simulink model "PassengerCar"  (R2019b)
settings: Solver=ode1  StartTime=0  StopTime=25  FixedStep=1.0000000000000000e-003  RelTol=1e-3
InitFcn:
  | sampleTime = str2double(get_param(bdroot, 'FixedStep'));
undefined symbols (not defined in the file or in its folder): AccPedalPos, BrakePedalPos, BrakeSwitch, DiscIntNeverNeededParam, DYNA4, EngSpd, IgnitionSwitch, InitialGear, InitialSpeed, IntendedEngTrq, LeftIndicator, MainBrakePress, MaxGear, MDL, MinGear, RefAcc, RefLane, RefLatPos, RefPath, RefPathCurv, RefSpd, RefSpdPreview, RefSpdRetrospect, RightIndicator, SteeringWheelAng, SteeringWheelTrq, UserDefinedRefValue, vm_const
libraries: UtilitiesLibrary x31, simulink x18, WheelSystemModules x13, LongitudinalControllerModules x13, LateralControllerModules x7, AnimationBusselectorModules x5, EnvironmentModules x5, BasicEngineControlModules x5, MiscellaneousControlModules x5, Animation3Modules x4, AuxiliariesModules x4, TireModules x4
(part 30 of 39)

== system PassengerCar/Vehicle/Drivetrain/DrivetrainPhysics/DrivetrainPhysicsInputs/InputFromWheelSystem ==
  fromWheelSystem : Inport
  TDBusSelector : BusSelector  OutputSignals=FrontLeft.Wheel.RotSpd[rad/s],FrontRight.Wheel.RotSpd[rad/s],RearLeft.Wheel.RotSpd[rad/s],RearRight.Wheel.RotSpd[rad/s],Rear2Left.Wheel.RotSpd[rad/s],Rear2Right.Wheel.RotSpd[rad/s],Rear3Left.Wheel.RotSpd[rad/s],Rear3Right.Wheel.RotSpd[rad/s]
  __TDD__WheelSystem.RotSpdFL[rad/s] : Demux  Outputs=[1]
  __TDD__WheelSystem.RotSpdFR[rad/s] : Demux  Outputs=[1]
  __TDD__WheelSystem.RotSpdR2L[rad/s] : Demux  Outputs=[1]
  __TDD__WheelSystem.RotSpdR2R[rad/s] : Demux  Outputs=[1]
  __TDD__WheelSystem.RotSpdR3L[rad/s] : Demux  Outputs=[1]
  __TDD__WheelSystem.RotSpdR3R[rad/s] : Demux  Outputs=[1]
  __TDD__WheelSystem.RotSpdRL[rad/s] : Demux  Outputs=[1]
  __TDD__WheelSystem.RotSpdRR[rad/s] : Demux  Outputs=[1]
  __TDO__WheelSystem : BusCreator  Inputs=8
  WheelSystem___UNIQUE_1 : Outport  Description=|  PortDimensions=[8]  VectorParamsAs1DForOutWhenUnconnected=off
      | <name>FrontLeft.Wheel.RotSpd[rad/s]</name>
      | <comment></comment>
  wires:
  fromWheelSystem/1 -> TDBusSelector/1
  TDBusSelector/1 -> __TDD__WheelSystem.RotSpdFL[rad/s]/1  "<RotSpd[rad/s]>"
  __TDD__WheelSystem.RotSpdFL[rad/s]/1 -> __TDO__WheelSystem/1  "RotSpdFL[rad/s]"
  TDBusSelector/2 -> __TDD__WheelSystem.RotSpdFR[rad/s]/1  "<RotSpd[rad/s]>"
  __TDD__WheelSystem.RotSpdFR[rad/s]/1 -> __TDO__WheelSystem/2  "RotSpdFR[rad/s]"
  TDBusSelector/3 -> __TDD__WheelSystem.RotSpdRL[rad/s]/1  "<RotSpd[rad/s]>"
  __TDD__WheelSystem.RotSpdRL[rad/s]/1 -> __TDO__WheelSystem/3  "RotSpdRL[rad/s]"
  TDBusSelector/4 -> __TDD__WheelSystem.RotSpdRR[rad/s]/1  "<RotSpd[rad/s]>"
  __TDD__WheelSystem.RotSpdRR[rad/s]/1 -> __TDO__WheelSystem/4  "RotSpdRR[rad/s]"
  TDBusSelector/5 -> __TDD__WheelSystem.RotSpdR2L[rad/s]/1  "<RotSpd[rad/s]>"
  __TDD__WheelSystem.RotSpdR2L[rad/s]/1 -> __TDO__WheelSystem/5  "RotSpdR2L[rad/s]"
  TDBusSelector/6 -> __TDD__WheelSystem.RotSpdR2R[rad/s]/1  "<RotSpd[rad/s]>"
  __TDD__WheelSystem.RotSpdR2R[rad/s]/1 -> __TDO__WheelSystem/6  "RotSpdR2R[rad/s]"
  TDBusSelector/7 -> __TDD__WheelSystem.RotSpdR3L[rad/s]/1  "<RotSpd[rad/s]>"
  __TDD__WheelSystem.RotSpdR3L[rad/s]/1 -> __TDO__WheelSystem/7  "RotSpdR3L[rad/s]"
  TDBusSelector/8 -> __TDD__WheelSystem.RotSpdR3R[rad/s]/1  "<RotSpd[rad/s]>"
  __TDD__WheelSystem.RotSpdR3R[rad/s]/1 -> __TDO__WheelSystem/8  "RotSpdR3R[rad/s]"
  __TDO__WheelSystem/1 -> WheelSystem___UNIQUE_1/1  "WheelSystem"

== system PassengerCar/Vehicle/Drivetrain/DrivetrainPhysics/DrivetrainPhysicsOutputs/ClutchOutput ==
  note: negative clutch torque accelerates driven plate
  ClutchStates : Inport
  ClutchOutput : Subsystem  Tag=TESIS DYNAware Interface Block  mask{NeedsUpdate=off, SignalInfo=|}
      mask SignalInfo=|
      | {
      |   "Version": "4.6",
      |   "MuxedOutputBusName": "Clutch",
      |   "MuxedInputBusName": "input",
      |   "MuxedInputSelected": false,
      |   "MuxedOutputSelected": true,
      |   "SignalData": [
      |     {
      |       "initialValue": "0.0",
      |       "name": "Trq[Nm]",
      |       "comment": "",
      |       "minString": "",
      |       "maxString": "",
      |       "width": 1,
      |       "dataType": 0,
      |       "signalType": 0,
      |       "createSignal": false,
      |       "outputName": "Trq[Nm]",
      |       "generateSignalAccessBlock": false,
      |       "accessId": "$(parentId).$(blockName).$(outputName)"
      |     },
      |     {
      |       "initialValue": "0.0",
      |       "name": "Pos[0_1]",
      |       "comment": "",
      |       "minString": "",
      |       "maxString": "",
      |       "width": 1,
      |       "dataType": 0,
      |       "signalType": 0,
      |       "createSignal": false,
      |       "outputName": "Pos[0_1]",
      |       "generateSignalAccessBlock": false,
      |       "accessId": "$(parentId).$(blockName).$(outputName)"
      |     }
      |   ]
      | }
      mask prompts: NeedsUpdate "Specify, if subsystem content needs to be updated"; SignalInfo "Signal Info (json)"
      mask help: DYNA4 Interface Block Version 4.6
      mask init:
      | blockName = get_param(gcbh, 'Name');
      | parentId = DYNA4.ModelHandling.AccessID.getFromHierarchy(gcbh);
      | TD.InterfaceBlock.ModelCallbacks.GenerateContent(gcb);
      settings: DeleteFcn=TD.InterfaceBlock.ModelCallbacks.CloseGUI( gcbh );  NameChangeFcn=TD.InterfaceBlock.ModelCallbacks.BlockRenamedHandler(gcbh);  OpenFcn=TD.InterfaceBlock.ModelCallbacks.OpenGUI( gcbh );  CloseFcn=TD.InterfaceBlock.ModelCallbacks.CloseGUI( gcbh );
      mask Display:
      | image('InterfaceBlock.png','center');
      | port_label('input',1, 'Trq[Nm]');
      | port_label('input',2, 'Pos[0_1]');
      | port_label('output',1, 'Clutch');
  Demux2 : Demux  Outputs=[1 1]
  Clutch : Outport  VectorParamsAs1DForOutWhenUnconnected=off
  wires:
  Demux2/2 -> ClutchOutput/2(Pos[0_1]___UNIQUE_1)
  ClutchStates/1 -> Demux2/1
  ClutchOutput/1(Clutch___UNIQUE_1) -> Clutch/1
  Demux2/1 -> ClutchOutput/1(Trq[Nm]___UNIQUE_1)

== system PassengerCar/Vehicle/Drivetrain/DrivetrainPhysics/DrivetrainPhysicsOutputs/DrivetrainPhysicsOutput ==
  EngSpd[rad/s]___UNIQUE_1 : Inport  Description=|  PortDimensions=[1]
      | <name>EngSpd[rad/s]</name>
      | <comment></comment>
  EngAcc[rad/s**2]___UNIQUE_1 : Inport  Description=|  Port=2  PortDimensions=[1]
      | <name>EngAcc[rad/s**2]</name>
      | <comment></comment>
  Clutch___UNIQUE_1 : Inport  Description=|  Port=3
      | <name>Clutch</name>
      | <comment></comment>
  Transmission___UNIQUE_1 : Inport  Description=|  Port=4
      | <name>Transmission</name>
      | <comment></comment>
  TransferCase___UNIQUE_1 : Inport  Description=|  Port=5
      | <name>TransferCase</name>
      | <comment></comment>
  FrontDifferential___UNIQUE_1 : Inport  Description=|  Port=6
      | <name>FrontDifferential</name>
      | <comment></comment>
  FrontLeftShaft___UNIQUE_1 : Inport  Description=|  Port=7
      | <name>FrontLeftShaft</name>
      | <comment></comment>
  FrontRightShaft___UNIQUE_1 : Inport  Description=|  Port=8
      | <name>FrontRightShaft</name>
      | <comment></comment>
  RearDifferential___UNIQUE_1 : Inport  Description=|  Port=9
      | <name>RearDifferential</name>
      | <comment></comment>
  RearLeftShaft___UNIQUE_1 : Inport  Description=|  Port=10
      | <name>RearLeftShaft</name>
      | <comment></comment>
  RearRightShaft___UNIQUE_1 : Inport  Description=|  Port=11
      | <name>RearRightShaft</name>
      | <comment></comment>
  Rear2Differential___UNIQUE_1 : Inport  Description=|  Port=12
      | <name>Rear2Differential</name>
      | <comment></comment>
  Rear2LeftShaft___UNIQUE_1 : Inport  Description=|  Port=13
      | <name>Rear2LeftShaft</name>
      | <comment></comment>
  Rear2RightShaft___UNIQUE_1 : Inport  Description=|  Port=14
      | <name>Rear2RightShaft</name>
      | <comment></comment>
  Rear3Differential___UNIQUE_1 : Inport  Description=|  Port=15
      | <name>Rear3Differential</name>
      | <comment></comment>
  Rear3LeftShaft___UNIQUE_1 : Inport  Description=|  Port=16
      | <name>Rear3LeftShaft</name>
      | <comment></comment>
  Rear3RightShaft___UNIQUE_1 : Inport  Description=|  Port=17
      | <name>Rear3RightShaft</name>
      | <comment></comment>
  TotalRatio[-]___UNIQUE_1 : Inport  Description=|  Port=18  PortDimensions=[1]
      | <name>TotalRatio[-]</name>
      | <comment></comment>
  __TDD__DrivetrainPhysics.EngAcc[rad/s**2] : Demux  Outputs=[1]
  __TDD__DrivetrainPhysics.EngSpd[rad/s] : Demux  Outputs=[1]
  __TDD__DrivetrainPhysics.TotalRatio[-] : Demux  Outputs=[1]
  __TDO__DrivetrainPhysics : BusCreator  Inputs=18
  DrivetrainPhysics___UNIQUE_1 : Outport  Description=|  VectorParamsAs1DForOutWhenUnconnected=off
      | <name>EngSpd[rad/s]</name>
      | <comment></comment>
  wires:
  EngSpd[rad/s]___UNIQUE_1/1 -> __TDD__DrivetrainPhysics.EngSpd[rad/s]/1
  __TDD__DrivetrainPhysics.EngSpd[rad/s]/1 -> __TDO__DrivetrainPhysics/1  "EngSpd[rad/s]"
  EngAcc[rad/s**2]___UNIQUE_1/1 -> __TDD__DrivetrainPhysics.EngAcc[rad/s**2]/1
  __TDD__DrivetrainPhysics.EngAcc[rad/s**2]/1 -> __TDO__DrivetrainPhysics/2  "EngAcc[rad/s**2]"
  Clutch___UNIQUE_1/1 -> __TDO__DrivetrainPhysics/3  "Clutch"
  Transmission___UNIQUE_1/1 -> __TDO__DrivetrainPhysics/4  "Transmission"
  TransferCase___UNIQUE_1/1 -> __TDO__DrivetrainPhysics/5  "TransferCase"
  FrontDifferential___UNIQUE_1/1 -> __TDO__DrivetrainPhysics/6  "FrontDifferential"
  FrontLeftShaft___UNIQUE_1/1 -> __TDO__DrivetrainPhysics/7  "FrontLeftShaft"
  FrontRightShaft___UNIQUE_1/1 -> __TDO__DrivetrainPhysics/8  "FrontRightShaft"
  RearDifferential___UNIQUE_1/1 -> __TDO__DrivetrainPhysics/9  "RearDifferential"
  RearLeftShaft___UNIQUE_1/1 -> __TDO__DrivetrainPhysics/10  "RearLeftShaft"
  RearRightShaft___UNIQUE_1/1 -> __TDO__DrivetrainPhysics/11  "RearRightShaft"
  Rear2Differential___UNIQUE_1/1 -> __TDO__DrivetrainPhysics/12  "Rear2Differential"
  Rear2LeftShaft___UNIQUE_1/1 -> __TDO__DrivetrainPhysics/13  "Rear2LeftShaft"
  Rear2RightShaft___UNIQUE_1/1 -> __TDO__DrivetrainPhysics/14  "Rear2RightShaft"
  Rear3Differential___UNIQUE_1/1 -> __TDO__DrivetrainPhysics/15  "Rear3Differential"
  Rear3LeftShaft___UNIQUE_1/1 -> __TDO__DrivetrainPhysics/16  "Rear3LeftShaft"
  Rear3RightShaft___UNIQUE_1/1 -> __TDO__DrivetrainPhysics/17  "Rear3RightShaft"
  TotalRatio[-]___UNIQUE_1/1 -> __TDD__DrivetrainPhysics.TotalRatio[-]/1
  __TDD__DrivetrainPhysics.TotalRatio[-]/1 -> __TDO__DrivetrainPhysics/18  "TotalRatio[-]"
  __TDO__DrivetrainPhysics/1 -> DrivetrainPhysics___UNIQUE_1/1  "DrivetrainPhysics"

== system PassengerCar/Vehicle/Drivetrain/DrivetrainPhysics/DrivetrainPhysicsOutputs/FrontDifferentialOutput ==
  In2 : Inport
  FrontDifferentialOutput : Subsystem  Tag=TESIS DYNAware Interface Block  mask{NeedsUpdate=off, SignalInfo=|}
      mask SignalInfo=|
      | {
      |   "Version": "4.6",
      |   "MuxedOutputBusName": "FrontDifferential",
      |   "MuxedInputBusName": "",
      |   "MuxedInputSelected": false,
      |   "MuxedOutputSelected": true,
      |   "SignalData": [
      |     {
      |       "initialValue": "0.0",
      |       "name": "InSpd[rad/s]",
      |       "comment": "",
      |       "minString": "",
      |       "maxString": "",
      |       "width": 1,
      |       "dataType": 0,
      |       "signalType": 0,
      |       "createSignal": false,
      |       "outputName": "InSpd[rad/s]",
      |       "generateSignalAccessBlock": false,
      |       "accessId": "$(parentId).$(blockName).$(outputName)"
      |     },
      |     {
      |       "initialValue": "0.0",
      |       "name": "LeftOutCutTrq[Nm]",
      |       "comment": "",
      |       "minString": "",
      |       "maxString": "",
      |       "width": 1,
      |       "dataType": 0,
      |       "signalType": 0,
      |       "createSignal": false,
      |       "outputName": "LeftOutCutTrq[Nm]",
      |       "generateSignalAccessBlock": false,
      |       "accessId": "$(parentId).$(blockName).$(outputName)"
      |     },
      |     {
      |       "initialValue": "0.0",
      |       "name": "RightOutCutTrq[Nm]",
      |       "comment": "",
      |       "minString": "",
      |       "maxString": "",
      |       "width": 1,
      |       "dataType": 0,
      |       "signalType": 0,
      |       "createSignal": false,
      |       "outputName": "RightOutCutTrq[Nm]",
      |       "generateSignalAccessBlock": false,
      |       "accessId": "$(parentId).$(blockName).$(outputName)"
      |     },
      |     {
      |       "initialValue": "0.0",
      |       "name": "LossPower[W]",
      |       "comment": "",
      |       "minString": "",
      |       "maxString": "",
      |       "width": 1,
      |       "dataType": 0,
      |       "signalType": 0,
      |       "createSignal": false,
      |       "outputName": "LossPower[W]",
      |       "generateSignalAccessBlock": false,
      |       "accessId": "$(parentId).$(blockName).$(outputName)"
      |     }
      |   ]
      | }
      mask prompts: NeedsUpdate "Specify, if subsystem content needs to be updated"; SignalInfo "Signal Info (json)"
      mask help: DYNA4 Interface Block Version 4.6
      mask init:
      | blockName = get_param(gcbh, 'Name');
      | parentId = DYNA4.ModelHandling.AccessID.getFromHierarchy(gcbh);
      | TD.InterfaceBlock.ModelCallbacks.GenerateContent(gcb);
      settings: DeleteFcn=TD.InterfaceBlock.ModelCallbacks.CloseGUI( gcbh );  NameChangeFcn=TD.InterfaceBlock.ModelCallbacks.BlockRenamedHandler(gcbh);  OpenFcn=TD.InterfaceBlock.ModelCallbacks.OpenGUI( gcbh );  CloseFcn=TD.InterfaceBlock.ModelCallbacks.CloseGUI( gcbh );
      mask Display:
      | image('InterfaceBlock.png','center');
      | port_label('input',1, 'InSpd[rad/s]');
      | port_label('input',2, 'LeftOutCutTrq[Nm]');
      | port_label('input',3, 'RightOutCutTrq[Nm]');
      | port_label('input',4, 'LossPower[W]');
      | port_label('output',1, 'FrontDifferential');
  zero : Constant  Value=0
  zero1 : Constant  Value=0
  zero2 : Constant  Value=0
  FrontDifferential : Outport  VectorParamsAs1DForOutWhenUnconnected=off
  wires:
  In2/1 -> FrontDifferentialOutput/1(InSpd[rad/s]___UNIQUE_1)
  FrontDifferentialOutput/1(FrontDifferential___UNIQUE_1) -> FrontDifferential/1
  zero/1 -> FrontDifferentialOutput/2(LeftOutCutTrq[Nm]___UNIQUE_1)
  zero2/1 -> FrontDifferentialOutput/4(LossPower[W]___UNIQUE_1)
  zero1/1 -> FrontDifferentialOutput/3(RightOutCutTrq[Nm]___UNIQUE_1)

== system PassengerCar/Vehicle/Drivetrain/DrivetrainPhysics/DrivetrainPhysicsOutputs/FrontLeftShaftOutput ==
  In1 : Inport
  Demux : Demux  Outputs=[1 1 1 1 1]
  FrontLeftShaftOutput : Subsystem  Tag=TESIS DYNAware Interface Block  mask{NeedsUpdate=off, SignalInfo=|}
      mask SignalInfo=|
      | {
      |   "Version": "4.6",
      |   "MuxedOutputBusName": "FrontLeftShaft",
      |   "MuxedInputBusName": "input",
      |   "MuxedInputSelected": false,
      |   "MuxedOutputSelected": true,
      |   "SignalData": [
      |     {
      |       "initialValue": "0.0",
      |       "name": "Trq[Nm]",
      |       "comment": "",
      |       "minString": "",
      |       "maxString": "",
      |       "width": 1,
      |       "dataType": 0,
      |       "signalType": 0,
      |       "createSignal": false,
      |       "outputName": "Trq[Nm]",
      |       "generateSignalAccessBlock": false,
      |       "accessId": "$(parentId).$(blockName).$(outputName)"
      |     },
      |     {
      |       "initialValue": "0.0",
      |       "name": "RotSpdDifferentialOut[rad/s]",
      |       "comment": "",
      |       "minString": "",
      |       "maxString": "",
      |       "width": 1,
      |       "dataType": 0,
      |       "signalType": 0,
      |       "createSignal": false,
      |       "outputName": "RotSpdDifferentialOut[rad/s]",
      |       "generateSignalAccessBlock": false,
      |       "accessId": "$(parentId).$(blockName).$(outputName)"
      |     },
      |     {
      |       "initialValue": "0.0",
      |       "name": "RotAcc[rad/s**2]",
      |       "comment": "",
      |       "minString": "",
      |       "maxString": "",
      |       "width": 1,
      |       "dataType": 0,
      |       "signalType": 0,
      |       "createSignal": false,
      |       "outputName": "RotAcc[rad/s**2]",
      |       "generateSignalAccessBlock": false,
      |       "accessId": "$(parentId).$(blockName).$(outputName)"
      |     },
      |     {
      |       "initialValue": "0.0",
      |       "name": "DerivativeOfTrq_wrt_RotAng[Nm/rad]",
      |       "comment": "",
      |       "minString": "",
      |       "maxString": "",
      |       "width": 1,
      |       "dataType": 0,
      |       "signalType": 0,
      |       "createSignal": false,
      |       "outputName": "DerivativeOfTrq_wrt_RotAng[Nm/rad]",
      |       "generateSignalAccessBlock": false,
      |       "accessId": "$(parentId).$(blockName).$(outputName)"
      |     },
      |     {
      |       "initialValue": "0.0",
      |       "name": "DerivativeOfTrq_wrt_WheelSpd[Nm/(rad/s)]",
      |       "comment": "",
      |       "minString": "",
      |       "maxString": "",
      |       "width": 1,
      |       "dataType": 0,
      |       "signalType": 0,
      |       "createSignal": false,
      |       "outputName": "DerivativeOfTrq_wrt_WheelSpd[Nm/(rad/s)]",
      |       "generateSignalAccessBlock": false,
      |       "accessId": "$(parentId).$(blockName).$(outputName)"
      |     },
      |     {
      |       "initialValue": "0.0",
      |       "name": "AddInrt[kg*m**2]",
      |       "comment": "",
      |       "minString": "",
      |       "maxString": "",
      |       "width": 1,
      |       "dataType": 0,
      |       "signalType": 0,
      |       "createSignal": false,
      |       "outputName": "AddInrt[kg*m**2]",
      |       "generateSignalAccessBlock": false,
      |       "accessId": "$(parentId).$(blockName).$(outputName)"
      |     },
      |     {
      |       "initialValue": "0.0",
      |       "name": "FrictionTrq[Nm]",
      |       "comment": "",
      |       "minString": "",
      |       "maxString": "",
      |       "width": 1,
      |       "dataType": 0,
      |       "signalType": 0,
      |       "createSignal": false,
      |       "outputName": "FrictionTrq[Nm]",
      |       "generateSignalAccessBlock": false,
      |       "accessId": "$(parentId).$(blockName).$(outputName)"
      |     }
      |   ]
      | }
      mask prompts: NeedsUpdate "Specify, if subsystem content needs to be updated"; SignalInfo "Signal Info (json)"
      mask help: DYNA4 Interface Block Version 4.6
      mask init:
      | blockName = get_param(gcbh, 'Name');
      | parentId = DYNA4.ModelHandling.AccessID.getFromHierarchy(gcbh);
      | TD.InterfaceBlock.ModelCallbacks.GenerateContent(gcb);
      settings: DeleteFcn=TD.InterfaceBlock.ModelCallbacks.CloseGUI( gcbh );  NameChangeFcn=TD.InterfaceBlock.ModelCallbacks.BlockRenamedHandler(gcbh);  OpenFcn=TD.InterfaceBlock.ModelCallbacks.OpenGUI( gcbh );  CloseFcn=TD.InterfaceBlock.ModelCallbacks.CloseGUI( gcbh );
      mask Display:
      | image('InterfaceBlock.png','center');
      | port_label('input',1, 'Trq[Nm]');
      | port_label('input',2, 'RotSpdDifferentialOut[rad/s]');
      | port_label('input',3, 'RotAcc[rad/s**2]');
      | port_label('input',4, 'DerivativeOfTrq_wrt_RotAng[Nm/rad]');
      | port_label('input',5, 'DerivativeOfTrq_wrt_WheelSpd[Nm/(rad/s)]');
      | port_label('input',6, 'AddInrt[kg*m**2]');
      | port_label('input',7, 'FrictionTrq[Nm]');
      | port_label('output',1, 'FrontLeftShaft');
  zero : Constant  Value=0
  zero1 : Constant  Value=0
  FrontLeftShaft : Outport  VectorParamsAs1DForOutWhenUnconnected=off
  wires:
  In1/1 -> Demux/1
  FrontLeftShaftOutput/1(FrontLeftShaft___UNIQUE_1) -> FrontLeftShaft/1
  Demux/3 -> FrontLeftShaftOutput/3(RotAcc[rad/s**2]___UNIQUE_1)
  zero1/1 -> FrontLeftShaftOutput/7(FrictionTrq[Nm]___UNIQUE_1)
  zero/1 -> FrontLeftShaftOutput/6(AddInrt[kg*m**2]___UNIQUE_1)
  Demux/5 -> FrontLeftShaftOutput/5(DerivativeOfTrq_wrt_WheelSpd[Nm/(rad/s)]___UNIQUE_1)
  Demux/4 -> FrontLeftShaftOutput/4(DerivativeOfTrq_wrt_RotAng[Nm/rad]___UNIQUE_1)
  Demux/2 -> FrontLeftShaftOutput/2(RotSpdDifferentialOut[rad/s]___UNIQUE_1)
  Demux/1 -> FrontLeftShaftOutput/1(Trq[Nm]___UNIQUE_1)

== system PassengerCar/Vehicle/Drivetrain/DrivetrainPhysics/DrivetrainPhysicsOutputs/FrontRightShaftOutput ==
  In1 : Inport
  Demux : Demux  Outputs=[1 1 1 1 1]
  FrontRightShaftOutput : Subsystem  Tag=TESIS DYNAware Interface Block  mask{NeedsUpdate=off, SignalInfo=|}
      mask SignalInfo=|
      | {
      |   "Version": "4.6",
      |   "MuxedOutputBusName": "FrontRightShaft",
      |   "MuxedInputBusName": "input",
      |   "MuxedInputSelected": false,
      |   "MuxedOutputSelected": true,
      |   "SignalData": [
      |     {
      |       "initialValue": "0.0",
      |       "name": "Trq[Nm]",
      |       "comment": "",
      |       "minString": "",
      |       "maxString": "",
      |       "width": 1,
      |       "dataType": 0,
      |       "signalType": 0,
      |       "createSignal": false,
      |       "outputName": "Trq[Nm]",
      |       "generateSignalAccessBlock": false,
      |       "accessId": "$(parentId).$(blockName).$(outputName)"
      |     },
      |     {
      |       "initialValue": "0.0",
      |       "name": "RotSpdDifferentialOut[rad/s]",
      |       "comment": "",
      |       "minString": "",
      |       "maxString": "",
      |       "width": 1,
      |       "dataType": 0,
      |       "signalType": 0,
      |       "createSignal": false,
      |       "outputName": "RotSpdDifferentialOut[rad/s]",
      |       "generateSignalAccessBlock": false,
      |       "accessId": "$(parentId).$(blockName).$(outputName)"
      |     },
      |     {
      |       "initialValue": "0.0",
      |       "name": "RotAcc[rad/s**2]",
      |       "comment": "",
      |       "minString": "",
      |       "maxString": "",
      |       "width": 1,
      |       "dataType": 0,
      |       "signalType": 0,
      |       "createSignal": false,
      |       "outputName": "RotAcc[rad/s**2]",
      |       "generateSignalAccessBlock": false,
      |       "accessId": "$(parentId).$(blockName).$(outputName)"
      |     },
      |     {
      |       "initialValue": "0.0",
      |       "name": "DerivativeOfTrq_wrt_RotAng[Nm/rad]",
      |       "comment": "",
      |       "minString": "",
      |       "maxString": "",
      |       "width": 1,
      |       "dataType": 0,
      |       "signalType": 0,
      |       "createSignal": false,
      |       "outputName": "DerivativeOfTrq_wrt_RotAng[Nm/rad]",
      |       "generateSignalAccessBlock": false,
      |       "accessId": "$(parentId).$(blockName).$(outputName)"
      |     },
      |     {
      |       "initialValue": "0.0",
      |       "name": "DerivativeOfTrq_wrt_WheelSpd[Nm/(rad/s)]",
      |       "comment": "",
      |       "minString": "",
      |       "maxString": "",
      |       "width": 1,
      |       "dataType": 0,
      |       "signalType": 0,
      |       "createSignal": false,
      |       "outputName": "DerivativeOfTrq_wrt_WheelSpd[Nm/(rad/s)]",
      |       "generateSignalAccessBlock": false,
      |       "accessId": "$(parentId).$(blockName).$(outputName)"
      |     },
      |     {
      |       "initialValue": "0.0",
      |       "name": "AddInrt[kg*m**2]",
      |       "comment": "",
      |       "minString": "",
      |       "maxString": "",
      |       "width": 1,
      |       "dataType": 0,
      |       "signalType": 0,
      |       "createSignal": false,
      |       "outputName": "AddInrt[kg*m**2]",
      |       "generateSignalAccessBlock": false,
      |       "accessId": "$(parentId).$(blockName).$(outputName)"
      |     },
      |     {
      |       "initialValue": "0.0",
      |       "name": "FrictionTrq[Nm]",
      |       "comment": "",
      |       "minString": "",
      |       "maxString": "",
      |       "width": 1,
      |       "dataType": 0,
      |       "signalType": 0,
      |       "createSignal": false,
      |       "outputName": "FrictionTrq[Nm]",
      |       "generateSignalAccessBlock": false,
      |       "accessId": "$(parentId).$(blockName).$(outputName)"
      |     }
      |   ]
      | }
      mask prompts: NeedsUpdate "Specify, if subsystem content needs to be updated"; SignalInfo "Signal Info (json)"
      mask help: DYNA4 Interface Block Version 4.6
      mask init:
      | blockName = get_param(gcbh, 'Name');
      | parentId = DYNA4.ModelHandling.AccessID.getFromHierarchy(gcbh);
      | TD.InterfaceBlock.ModelCallbacks.GenerateContent(gcb);
      settings: DeleteFcn=TD.InterfaceBlock.ModelCallbacks.CloseGUI( gcbh );  NameChangeFcn=TD.InterfaceBlock.ModelCallbacks.BlockRenamedHandler(gcbh);  OpenFcn=TD.InterfaceBlock.ModelCallbacks.OpenGUI( gcbh );  CloseFcn=TD.InterfaceBlock.ModelCallbacks.CloseGUI( gcbh );
      mask Display:
      | image('InterfaceBlock.png','center');
      | port_label('input',1, 'Trq[Nm]');
      | port_label('input',2, 'RotSpdDifferentialOut[rad/s]');
      | port_label('input',3, 'RotAcc[rad/s**2]');
      | port_label('input',4, 'DerivativeOfTrq_wrt_RotAng[Nm/rad]');
      | port_label('input',5, 'DerivativeOfTrq_wrt_WheelSpd[Nm/(rad/s)]');
      | port_label('input',6, 'AddInrt[kg*m**2]');
      | port_label('input',7, 'FrictionTrq[Nm]');
      | port_label('output',1, 'FrontRightShaft');
  zero : Constant  Value=0
  zero1 : Constant  Value=0
  FrontRightShaft : Outport  VectorParamsAs1DForOutWhenUnconnected=off
  wires:
  Demux/1 -> FrontRightShaftOutput/1(Trq[Nm]___UNIQUE_1)
  Demux/2 -> FrontRightShaftOutput/2(RotSpdDifferentialOut[rad/s]___UNIQUE_1)
  Demux/4 -> FrontRightShaftOutput/4(DerivativeOfTrq_wrt_RotAng[Nm/rad]___UNIQUE_1)
  Demux/5 -> FrontRightShaftOutput/5(DerivativeOfTrq_wrt_WheelSpd[Nm/(rad/s)]___UNIQUE_1)
  zero/1 -> FrontRightShaftOutput/6(AddInrt[kg*m**2]___UNIQUE_1)
  zero1/1 -> FrontRightShaftOutput/7(FrictionTrq[Nm]___UNIQUE_1)
  Demux/3 -> FrontRightShaftOutput/3(RotAcc[rad/s**2]___UNIQUE_1)
  FrontRightShaftOutput/1(FrontRightShaft___UNIQUE_1) -> FrontRightShaft/1
  In1/1 -> Demux/1

== system PassengerCar/Vehicle/Drivetrain/DrivetrainPhysics/DrivetrainPhysicsOutputs/Rear2DifferentialOutput ==
  In2 : Inport
  Rear2DifferentialOutput : Subsystem  Tag=TESIS DYNAware Interface Block  mask{NeedsUpdate=off, SignalInfo=|}
      mask SignalInfo=|
      | {
      |   "Version": "4.6",
      |   "MuxedOutputBusName": "Rear2Differential",
      |   "MuxedInputBusName": "",
      |   "MuxedInputSelected": false,
      |   "MuxedOutputSelected": true,
      |   "SignalData": [
      |     {
      |       "initialValue": "0.0",
      |       "name": "InSpd[rad/s]",
      |       "comment": "",
      |       "minString": "",
      |       "maxString": "",
      |       "width": 1,
      |       "dataType": 0,
      |       "signalType": 0,
      |       "createSignal": false,
      |       "outputName": "InSpd[rad/s]",
      |       "generateSignalAccessBlock": false,
      |       "accessId": "$(parentId).$(blockName).$(outputName)"
      |     },
      |     {
      |       "initialValue": "0.0",
      |       "name": "LeftOutCutTrq[Nm]",
      |       "comment": "",
      |       "minString": "",
      |       "maxString": "",
      |       "width": 1,
      |       "dataType": 0,
      |       "signalType": 0,
      |       "createSignal": false,
      |       "outputName": "LeftOutCutTrq[Nm]",
      |       "generateSignalAccessBlock": false,
      |       "accessId": "$(parentId).$(blockName).$(outputName)"
      |     },
      |     {
      |       "initialValue": "0.0",
      |       "name": "RightOutCutTrq[Nm]",
      |       "comment": "",
      |       "minString": "",
      |       "maxString": "",
      |       "width": 1,
      |       "dataType": 0,
      |       "signalType": 0,
      |       "createSignal": false,
      |       "outputName": "RightOutCutTrq[Nm]",
      |       "generateSignalAccessBlock": false,
      |       "accessId": "$(parentId).$(blockName).$(outputName)"
      |     },
      |     {
      |       "initialValue": "0.0",
      |       "name": "LossPower[W]",
      |       "comment": "",
      |       "minString": "",
      |       "maxString": "",
      |       "width": 1,
      |       "dataType": 0,
      |       "signalType": 0,
      |       "createSignal": false,
      |       "outputName": "LossPower[W]",
      |       "generateSignalAccessBlock": false,
      |       "accessId": "$(parentId).$(blockName).$(outputName)"
      |     }
      |   ]
      | }
      mask prompts: NeedsUpdate "Specify, if subsystem content needs to be updated"; SignalInfo "Signal Info (json)"
      mask help: DYNA4 Interface Block Version 4.6
      mask init:
      | blockName = get_param(gcbh, 'Name');
      | parentId = DYNA4.ModelHandling.AccessID.getFromHierarchy(gcbh);
      | TD.InterfaceBlock.ModelCallbacks.GenerateContent(gcb);
      settings: DeleteFcn=TD.InterfaceBlock.ModelCallbacks.CloseGUI( gcbh );  NameChangeFcn=TD.InterfaceBlock.ModelCallbacks.BlockRenamedHandler(gcbh);  OpenFcn=TD.InterfaceBlock.ModelCallbacks.OpenGUI( gcbh );  CloseFcn=TD.InterfaceBlock.ModelCallbacks.CloseGUI( gcbh );
      mask Display:
      | image('InterfaceBlock.png','center');
      | port_label('input',1, 'InSpd[rad/s]');
      | port_label('input',2, 'LeftOutCutTrq[Nm]');
      | port_label('input',3, 'RightOutCutTrq[Nm]');
      | port_label('input',4, 'LossPower[W]');
      | port_label('output',1, 'Rear2Differential');
  zero : Constant  Value=0
  zero1 : Constant  Value=0
  zero2 : Constant  Value=0
  Rear2Differential : Outport  VectorParamsAs1DForOutWhenUnconnected=off
  wires:
  In2/1 -> Rear2DifferentialOutput/1(InSpd[rad/s]___UNIQUE_1)
  Rear2DifferentialOutput/1(Rear2Differential___UNIQUE_1) -> Rear2Differential/1
  zero/1 -> Rear2DifferentialOutput/2(LeftOutCutTrq[Nm]___UNIQUE_1)
  zero2/1 -> Rear2DifferentialOutput/4(LossPower[W]___UNIQUE_1)
  zero1/1 -> Rear2DifferentialOutput/3(RightOutCutTrq[Nm]___UNIQUE_1)

== system PassengerCar/Vehicle/Drivetrain/DrivetrainPhysics/DrivetrainPhysicsOutputs/Rear2LeftShaftOutput ==
  In1 : Inport
  Demux : Demux  Outputs=[1 1 1 1 1]
  Rear2LeftShaftOutput : Subsystem  Tag=TESIS DYNAware Interface Block  mask{NeedsUpdate=off, SignalInfo=|}
      mask SignalInfo=|
      | {
      |   "Version": "4.6",
      |   "MuxedOutputBusName": "Rear2LeftShaft",
      |   "MuxedInputBusName": "input",
      |   "MuxedInputSelected": false,
      |   "MuxedOutputSelected": true,
      |   "SignalData": [
      |     {
      |       "initialValue": "0.0",
      |       "name": "Trq[Nm]",
      |       "comment": "",
      |       "minString": "",
      |       "maxString": "",
      |       "width": 1,
      |       "dataType": 0,
      |       "signalType": 0,
      |       "createSignal": false,
      |       "outputName": "Trq[Nm]",
      |       "generateSignalAccessBlock": false,
      |       "accessId": "$(parentId).$(blockName).$(outputName)"
      |     },
      |     {
      |       "initialValue": "0.0",
      |       "name": "RotSpdDifferentialOut[rad/s]",
      |       "comment": "",
      |       "minString": "",
      |       "maxString": "",
      |       "width": 1,
      |       "dataType": 0,
      |       "signalType": 0,
      |       "createSignal": false,
      |       "outputName": "RotSpdDifferentialOut[rad/s]",
      |       "generateSignalAccessBlock": false,
      |       "accessId": "$(parentId).$(blockName).$(outputName)"
      |     },
      |     {
      |       "initialValue": "0.0",
      |       "name": "RotAcc[rad/s**2]",
      |       "comment": "",
      |       "minString": "",
      |       "maxString": "",
      |       "width": 1,
      |       "dataType": 0,
      |       "signalType": 0,
      |       "createSignal": false,
      |       "outputName": "RotAcc[rad/s**2]",
      |       "generateSignalAccessBlock": false,
      |       "accessId": "$(parentId).$(blockName).$(outputName)"
      |     },
      |     {
      |       "initialValue": "0.0",
      |       "name": "DerivativeOfTrq_wrt_RotAng[Nm/rad]",
      |       "comment": "",
      |       "minString": "",
      |       "maxString": "",
      |       "width": 1,
      |       "dataType": 0,
      |       "signalType": 0,
      |       "createSignal": false,
      |       "outputName": "DerivativeOfTrq_wrt_RotAng[Nm/rad]",
      |       "generateSignalAccessBlock": false,
      |       "accessId": "$(parentId).$(blockName).$(outputName)"
      |     },
      |     {
      |       "initialValue": "0.0",
      |       "name": "DerivativeOfTrq_wrt_WheelSpd[Nm/(rad/s)]",
      |       "comment": "",
      |       "minString": "",
      |       "maxString": "",
      |       "width": 1,
      |       "dataType": 0,
      |       "signalType": 0,
      |       "createSignal": false,
      |       "outputName": "DerivativeOfTrq_wrt_WheelSpd[Nm/(rad/s)]",
      |       "generateSignalAccessBlock": false,
      |       "accessId": "$(parentId).$(blockName).$(outputName)"
      |     },
      |     {
      |       "initialValue": "0.0",
      |       "name": "AddInrt[kg*m**2]",
      |       "comment": "",
      |       "minString": "",
      |       "maxString": "",
      |       "width": 1,
      |       "dataType": 0,
      |       "signalType": 0,
      |       "createSignal": false,
      |       "outputName": "AddInrt[kg*m**2]",
      |       "generateSignalAccessBlock": false,
      |       "accessId": "$(parentId).$(blockName).$(outputName)"
      |     },
      |     {
      |       "initialValue": "0.0",
      |       "name": "FrictionTrq[Nm]",
      |       "comment": "",
      |       "minString": "",
      |       "maxString": "",
      |       "width": 1,
      |       "dataType": 0,
      |       "signalType": 0,
      |       "createSignal": false,
      |       "outputName": "FrictionTrq[Nm]",
      |       "generateSignalAccessBlock": false,
      |       "accessId": "$(parentId).$(blockName).$(outputName)"
      |     }
      |   ]
      | }
      mask prompts: NeedsUpdate "Specify, if subsystem content needs to be updated"; SignalInfo "Signal Info (json)"
      mask help: DYNA4 Interface Block Version 4.6
      mask init:
      | blockName = get_param(gcbh, 'Name');
      | parentId = DYNA4.ModelHandling.AccessID.getFromHierarchy(gcbh);
      | TD.InterfaceBlock.ModelCallbacks.GenerateContent(gcb);
      settings: DeleteFcn=TD.InterfaceBlock.ModelCallbacks.CloseGUI( gcbh );  NameChangeFcn=TD.InterfaceBlock.ModelCallbacks.BlockRenamedHandler(gcbh);  OpenFcn=TD.InterfaceBlock.ModelCallbacks.OpenGUI( gcbh );  CloseFcn=TD.InterfaceBlock.ModelCallbacks.CloseGUI( gcbh );
      mask Display:
      | image('InterfaceBlock.png','center');
      | port_label('input',1, 'Trq[Nm]');
      | port_label('input',2, 'RotSpdDifferentialOut[rad/s]');
      | port_label('input',3, 'RotAcc[rad/s**2]');
      | port_label('input',4, 'DerivativeOfTrq_wrt_RotAng[Nm/rad]');
      | port_label('input',5, 'DerivativeOfTrq_wrt_WheelSpd[Nm/(rad/s)]');
      | port_label('input',6, 'AddInrt[kg*m**2]');
      | port_label('input',7, 'FrictionTrq[Nm]');
      | port_label('output',1, 'Rear2LeftShaft');
  zero : Constant  Value=0
  zero1 : Constant  Value=0
  Rear2LeftShaft : Outport  VectorParamsAs1DForOutWhenUnconnected=off
  wires:
  Demux/1 -> Rear2LeftShaftOutput/1(Trq[Nm]___UNIQUE_1)
  Demux/2 -> Rear2LeftShaftOutput/2(RotSpdDifferentialOut[rad/s]___UNIQUE_1)
  Demux/4 -> Rear2LeftShaftOutput/4(DerivativeOfTrq_wrt_RotAng[Nm/rad]___UNIQUE_1)
  Demux/5 -> Rear2LeftShaftOutput/5(DerivativeOfTrq_wrt_WheelSpd[Nm/(rad/s)]___UNIQUE_1)
  zero/1 -> Rear2LeftShaftOutput/6(AddInrt[kg*m**2]___UNIQUE_1)
  zero1/1 -> Rear2LeftShaftOutput/7(FrictionTrq[Nm]___UNIQUE_1)
  Demux/3 -> Rear2LeftShaftOutput/3(RotAcc[rad/s**2]___UNIQUE_1)
  Rear2LeftShaftOutput/1(Rear2LeftShaft___UNIQUE_1) -> Rear2LeftShaft/1
  In1/1 -> Demux/1

== system PassengerCar/Vehicle/Drivetrain/DrivetrainPhysics/DrivetrainPhysicsOutputs/Rear2RightShaftOutput ==
  In1 : Inport
  Demux : Demux  Outputs=[1 1 1 1 1]
  Rear2RightShaftOutput : Subsystem  Tag=TESIS DYNAware Interface Block  mask{NeedsUpdate=off, SignalInfo=|}
      mask SignalInfo=|
      | {
      |   "Version": "4.6",
      |   "MuxedOutputBusName": "Rear2RightShaft",
      |   "MuxedInputBusName": "input",
      |   "MuxedInputSelected": false,
      |   "MuxedOutputSelected": true,
      |   "SignalData": [
      |     {
      |       "initialValue": "0.0",
      |       "name": "Trq[Nm]",
      |       "comment": "",
      |       "minString": "",
      |       "maxString": "",
      |       "width": 1,
      |       "dataType": 0,
      |       "signalType": 0,
      |       "createSignal": false,
      |       "outputName": "Trq[Nm]",
      |       "generateSignalAccessBlock": false,
      |       "accessId": "$(parentId).$(blockName).$(outputName)"
      |     },
      |     {
      |       "initialValue": "0.0",
      |       "name": "RotSpdDifferentialOut[rad/s]",
      |       "comment": "",
      |       "minString": "",
      |       "maxString": "",
      |       "width": 1,
      |       "dataType": 0,
      |       "signalType": 0,
      |       "createSignal": false,
      |       "outputName": "RotSpdDifferentialOut[rad/s]",
      |       "generateSignalAccessBlock": false,
      |       "accessId": "$(parentId).$(blockName).$(outputName)"
      |     },
      |     {
      |       "initialValue": "0.0",
      |       "name": "RotAcc[rad/s**2]",
      |       "comment": "",
      |       "minString": "",
      |       "maxString": "",
      |       "width": 1,
      |       "dataType": 0,
      |       "signalType": 0,
      |       "createSignal": false,
      |       "outputName": "RotAcc[rad/s**2]",
      |       "generateSignalAccessBlock": false,
      |       "accessId": "$(parentId).$(blockName).$(outputName)"
      |     },
      |     {
      |       "initialValue": "0.0",
      |       "name": "DerivativeOfTrq_wrt_RotAng[Nm/rad]",
      |       "comment": "",
      |       "minString": "",
      |       "maxString": "",
      |       "width": 1,
      |       "dataType": 0,
      |       "signalType": 0,
      |       "createSignal": false,
      |       "outputName": "DerivativeOfTrq_wrt_RotAng[Nm/rad]",
      |       "generateSignalAccessBlock": false,
      |       "accessId": "$(parentId).$(blockName).$(outputName)"
      |     },
      |     {
      |       "initialValue": "0.0",
      |       "name": "DerivativeOfTrq_wrt_WheelSpd[Nm/(rad/s)]",
      |       "comment": "",
      |       "minString": "",
      |       "maxString": "",
      |       "width": 1,
      |       "dataType": 0,
      |       "signalType": 0,
      |       "createSignal": false,
      |       "outputName": "DerivativeOfTrq_wrt_WheelSpd[Nm/(rad/s)]",
      |       "generateSignalAccessBlock": false,
      |       "accessId": "$(parentId).$(blockName).$(outputName)"
      |     },
      |     {
      |       "initialValue": "0.0",
      |       "name": "AddInrt[kg*m**2]",
      |       "comment": "",
      |       "minString": "",
      |       "maxString": "",
      |       "width": 1,
      |       "dataType": 0,
      |       "signalType": 0,
      |       "createSignal": false,
      |       "outputName": "AddInrt[kg*m**2]",
      |       "generateSignalAccessBlock": false,
      |       "accessId": "$(parentId).$(blockName).$(outputName)"
      |     },
      |     {
      |       "initialValue": "0.0",
      |       "name": "FrictionTrq[Nm]",
      |       "comment": "",
      |       "minString": "",
      |       "maxString": "",
      |       "width": 1,
      |       "dataType": 0,
      |       "signalType": 0,
      |       "createSignal": false,
      |       "outputName": "FrictionTrq[Nm]",
      |       "generateSignalAccessBlock": false,
      |       "accessId": "$(parentId).$(blockName).$(outputName)"
      |     }
      |   ]
      | }
      mask prompts: NeedsUpdate "Specify, if subsystem content needs to be updated"; SignalInfo "Signal Info (json)"
      mask help: DYNA4 Interface Block Version 4.6
      mask init:
      | blockName = get_param(gcbh, 'Name');
      | parentId = DYNA4.ModelHandling.AccessID.getFromHierarchy(gcbh);
      | TD.InterfaceBlock.ModelCallbacks.GenerateContent(gcb);
      settings: DeleteFcn=TD.InterfaceBlock.ModelCallbacks.CloseGUI( gcbh );  NameChangeFcn=TD.InterfaceBlock.ModelCallbacks.BlockRenamedHandler(gcbh);  OpenFcn=TD.InterfaceBlock.ModelCallbacks.OpenGUI( gcbh );  CloseFcn=TD.InterfaceBlock.ModelCallbacks.CloseGUI( gcbh );
      mask Display:
      | image('InterfaceBlock.png','center');
      | port_label('input',1, 'Trq[Nm]');
      | port_label('input',2, 'RotSpdDifferentialOut[rad/s]');
      | port_label('input',3, 'RotAcc[rad/s**2]');
      | port_label('input',4, 'DerivativeOfTrq_wrt_RotAng[Nm/rad]');
      | port_label('input',5, 'DerivativeOfTrq_wrt_WheelSpd[Nm/(rad/s)]');
      | port_label('input',6, 'AddInrt[kg*m**2]');
      | port_label('input',7, 'FrictionTrq[Nm]');
      | port_label('output',1, 'Rear2RightShaft');
  zero : Constant  Value=0
  zero1 : Constant  Value=0
  Rear2RightShaft : Outport  VectorParamsAs1DForOutWhenUnconnected=off
  wires:
  In1/1 -> Demux/1
  Rear2RightShaftOutput/1(Rear2RightShaft___UNIQUE_1) -> Rear2RightShaft/1
  Demux/3 -> Rear2RightShaftOutput/3(RotAcc[rad/s**2]___UNIQUE_1)
  zero1/1 -> Rear2RightShaftOutput/7(FrictionTrq[Nm]___UNIQUE_1)
  zero/1 -> Rear2RightShaftOutput/6(AddInrt[kg*m**2]___UNIQUE_1)
  Demux/5 -> Rear2RightShaftOutput/5(DerivativeOfTrq_wrt_WheelSpd[Nm/(rad/s)]___UNIQUE_1)
  Demux/4 -> Rear2RightShaftOutput/4(DerivativeOfTrq_wrt_RotAng[Nm/rad]___UNIQUE_1)
  Demux/2 -> Rear2RightShaftOutput/2(RotSpdDifferentialOut[rad/s]___UNIQUE_1)
  Demux/1 -> Rear2RightShaftOutput/1(Trq[Nm]___UNIQUE_1)

== system PassengerCar/Vehicle/Drivetrain/DrivetrainPhysics/DrivetrainPhysicsOutputs/Rear3DifferentialOutput ==
  In2 : Inport
  Rear3DifferentialOutput : Subsystem  Tag=TESIS DYNAware Interface Block  mask{NeedsUpdate=off, SignalInfo=|}
      mask SignalInfo=|
      | {
      |   "Version": "4.6",
      |   "MuxedOutputBusName": "Rear3Differential",
      |   "MuxedInputBusName": "",
      |   "MuxedInputSelected": false,
      |   "MuxedOutputSelected": true,
      |   "SignalData": [
      |     {
      |       "initialValue": "0.0",
      |       "name": "InSpd[rad/s]",
      |       "comment": "",
      |       "minString": "",
      |       "maxString": "",
      |       "width": 1,
      |       "dataType": 0,
      |       "signalType": 0,
      |       "createSignal": false,
      |       "outputName": "InSpd[rad/s]",
      |       "generateSignalAccessBlock": false,
      |       "accessId": "$(parentId).$(blockName).$(outputName)"
      |     },
      |     {
      |       "initialValue": "0.0",
      |       "name": "LeftOutCutTrq[Nm]",
      |       "comment": "",
      |       "minString": "",
      |       "maxString": "",
      |       "width": 1,
      |       "dataType": 0,
      |       "signalType": 0,
      |       "createSignal": false,
      |       "outputName": "LeftOutCutTrq[Nm]",
      |       "generateSignalAccessBlock": false,
      |       "accessId": "$(parentId).$(blockName).$(outputName)"
      |     },
      |     {
      |       "initialValue": "0.0",
      |       "name": "RightOutCutTrq[Nm]",
      |       "comment": "",
      |       "minString": "",
      |       "maxString": "",
      |       "width": 1,
      |       "dataType": 0,
      |       "signalType": 0,
      |       "createSignal": false,
      |       "outputName": "RightOutCutTrq[Nm]",
      |       "generateSignalAccessBlock": false,
      |       "accessId": "$(parentId).$(blockName).$(outputName)"
      |     },
      |     {
      |       "initialValue": "0.0",
      |       "name": "LossPower[W]",
      |       "comment": "",
      |       "minString": "",
      |       "maxString": "",
      |       "width": 1,
      |       "dataType": 0,
      |       "signalType": 0,
      |       "createSignal": false,
      |       "outputName": "LossPower[W]",
      |       "generateSignalAccessBlock": false,
      |       "accessId": "$(parentId).$(blockName).$(outputName)"
      |     }
      |   ]
      | }
      mask prompts: NeedsUpdate "Specify, if subsystem content needs to be updated"; SignalInfo "Signal Info (json)"
      mask help: DYNA4 Interface Block Version 4.6
      mask init:
      | blockName = get_param(gcbh, 'Name');
      | parentId = DYNA4.ModelHandling.AccessID.getFromHierarchy(gcbh);
      | TD.InterfaceBlock.ModelCallbacks.GenerateContent(gcb);
      settings: DeleteFcn=TD.InterfaceBlock.ModelCallbacks.CloseGUI( gcbh );  NameChangeFcn=TD.InterfaceBlock.ModelCallbacks.BlockRenamedHandler(gcbh);  OpenFcn=TD.InterfaceBlock.ModelCallbacks.OpenGUI( gcbh );  CloseFcn=TD.InterfaceBlock.ModelCallbacks.CloseGUI( gcbh );
      mask Display:
      | image('InterfaceBlock.png','center');
      | port_label('input',1, 'InSpd[rad/s]');
      | port_label('input',2, 'LeftOutCutTrq[Nm]');
      | port_label('input',3, 'RightOutCutTrq[Nm]');
      | port_label('input',4, 'LossPower[W]');
      | port_label('output',1, 'Rear3Differential');
  zero : Constant  Value=0
  zero1 : Constant  Value=0
  zero2 : Constant  Value=0
  Rear3Differential : Outport  VectorParamsAs1DForOutWhenUnconnected=off
  wires:
  zero1/1 -> Rear3DifferentialOutput/3(RightOutCutTrq[Nm]___UNIQUE_1)
  zero2/1 -> Rear3DifferentialOutput/4(LossPower[W]___UNIQUE_1)
  zero/1 -> Rear3DifferentialOutput/2(LeftOutCutTrq[Nm]___UNIQUE_1)
  Rear3DifferentialOutput/1(Rear3Differential___UNIQUE_1) -> Rear3Differential/1
  In2/1 -> Rear3DifferentialOutput/1(InSpd[rad/s]___UNIQUE_1)

== system PassengerCar/Vehicle/Drivetrain/DrivetrainPhysics/DrivetrainPhysicsOutputs/Rear3LeftShaftOutput ==
  In1 : Inport
  Demux : Demux  Outputs=[1 1 1 1 1]
  Rear3LeftShaftOutput : Subsystem  Tag=TESIS DYNAware Interface Block  mask{NeedsUpdate=off, SignalInfo=|}
      mask SignalInfo=|
      | {
      |   "Version": "4.6",
      |   "MuxedOutputBusName": "Rear3LeftShaft",
      |   "MuxedInputBusName": "input",
      |   "MuxedInputSelected": false,
      |   "MuxedOutputSelected": true,
      |   "SignalData": [
      |     {
      |       "initialValue": "0.0",
      |       "name": "Trq[Nm]",
      |       "comment": "",
      |       "minString": "",
      |       "maxString": "",
      |       "width": 1,
      |       "dataType": 0,
      |       "signalType": 0,
      |       "createSignal": false,
      |       "outputName": "Trq[Nm]",
      |       "generateSignalAccessBlock": false,
      |       "accessId": "$(parentId).$(blockName).$(outputName)"
      |     },
      |     {
      |       "initialValue": "0.0",
      |       "name": "RotSpdDifferentialOut[rad/s]",
      |       "comment": "",
      |       "minString": "",
      |       "maxString": "",
      |       "width": 1,
      |       "dataType": 0,
      |       "signalType": 0,
      |       "createSignal": false,
      |       "outputName": "RotSpdDifferentialOut[rad/s]",
      |       "generateSignalAccessBlock": false,
      |       "accessId": "$(parentId).$(blockName).$(outputName)"
      |     },
      |     {
      |       "initialValue": "0.0",
      |       "name": "RotAcc[rad/s**2]",
      |       "comment": "",
      |       "minString": "",
      |       "maxString": "",
      |       "width": 1,
      |       "dataType": 0,
      |       "signalType": 0,
      |       "createSignal": false,
      |       "outputName": "RotAcc[rad/s**2]",
      |       "generateSignalAccessBlock": false,
      |       "accessId": "$(parentId).$(blockName).$(outputName)"
      |     },
      |     {
      |       "initialValue": "0.0",
      |       "name": "DerivativeOfTrq_wrt_RotAng[Nm/rad]",
      |       "comment": "",
      |       "minString": "",
      |       "maxString": "",
      |       "width": 1,
      |       "dataType": 0,
      |       "signalType": 0,
      |       "createSignal": false,
      |       "outputName": "DerivativeOfTrq_wrt_RotAng[Nm/rad]",
      |       "generateSignalAccessBlock": false,
      |       "accessId": "$(parentId).$(blockName).$(outputName)"
      |     },
      |     {
      |       "initialValue": "0.0",
      |       "name": "DerivativeOfTrq_wrt_WheelSpd[Nm/(rad/s)]",
      |       "comment": "",
      |       "minString": "",
      |       "maxString": "",
      |       "width": 1,
      |       "dataType": 0,
      |       "signalType": 0,
      |       "createSignal": false,
      |       "outputName": "DerivativeOfTrq_wrt_WheelSpd[Nm/(rad/s)]",
      |       "generateSignalAccessBlock": false,
      |       "accessId": "$(parentId).$(blockName).$(outputName)"
      |     },
      |     {
      |       "initialValue": "0.0",
      |       "name": "AddInrt[kg*m**2]",
      |       "comment": "",
      |       "minString": "",
      |       "maxString": "",
      |       "width": 1,
      |       "dataType": 0,
      |       "signalType": 0,
      |       "createSignal": false,
      |       "outputName": "AddInrt[kg*m**2]",
      |       "generateSignalAccessBlock": false,
      |       "accessId": "$(parentId).$(blockName).$(outputName)"
      |     },
      |     {
      |       "initialValue": "0.0",
      |       "name": "FrictionTrq[Nm]",
      |       "comment": "",
      |       "minString": "",
      |       "maxString": "",
      |       "width": 1,
      |       "dataType": 0,
      |       "signalType": 0,
      |       "createSignal": false,
      |       "outputName": "FrictionTrq[Nm]",
      |       "generateSignalAccessBlock": false,
      |       "accessId": "$(parentId).$(blockName).$(outputName)"
      |     }
      |   ]
      | }
      mask prompts: NeedsUpdate "Specify, if subsystem content needs to be updated"; SignalInfo "Signal Info (json)"
      mask help: DYNA4 Interface Block Version 4.6
      mask init:
      | blockName = get_param(gcbh, 'Name');
      | parentId = DYNA4.ModelHandling.AccessID.getFromHierarchy(gcbh);
      | TD.InterfaceBlock.ModelCallbacks.GenerateContent(gcb);
      settings: DeleteFcn=TD.InterfaceBlock.ModelCallbacks.CloseGUI( gcbh );  NameChangeFcn=TD.InterfaceBlock.ModelCallbacks.BlockRenamedHandler(gcbh);  OpenFcn=TD.InterfaceBlock.ModelCallbacks.OpenGUI( gcbh );  CloseFcn=TD.InterfaceBlock.ModelCallbacks.CloseGUI( gcbh );
      mask Display:
      | image('InterfaceBlock.png','center');
      | port_label('input',1, 'Trq[Nm]');
      | port_label('input',2, 'RotSpdDifferentialOut[rad/s]');
      | port_label('input',3, 'RotAcc[rad/s**2]');
      | port_label('input',4, 'DerivativeOfTrq_wrt_RotAng[Nm/rad]');
      | port_label('input',5, 'DerivativeOfTrq_wrt_WheelSpd[Nm/(rad/s)]');
      | port_label('input',6, 'AddInrt[kg*m**2]');
      | port_label('input',7, 'FrictionTrq[Nm]');
      | port_label('output',1, 'Rear3LeftShaft');
  zero : Constant  Value=0
  zero1 : Constant  Value=0
  Rear3LeftShaft : Outport  VectorParamsAs1DForOutWhenUnconnected=off
  wires:
  In1/1 -> Demux/1
  Rear3LeftShaftOutput/1(Rear3LeftShaft___UNIQUE_1) -> Rear3LeftShaft/1
  Demux/3 -> Rear3LeftShaftOutput/3(RotAcc[rad/s**2]___UNIQUE_1)
  zero1/1 -> Rear3LeftShaftOutput/7(FrictionTrq[Nm]___UNIQUE_1)
  zero/1 -> Rear3LeftShaftOutput/6(AddInrt[kg*m**2]___UNIQUE_1)
  Demux/5 -> Rear3LeftShaftOutput/5(DerivativeOfTrq_wrt_WheelSpd[Nm/(rad/s)]___UNIQUE_1)
  Demux/4 -> Rear3LeftShaftOutput/4(DerivativeOfTrq_wrt_RotAng[Nm/rad]___UNIQUE_1)
  Demux/2 -> Rear3LeftShaftOutput/2(RotSpdDifferentialOut[rad/s]___UNIQUE_1)
  Demux/1 -> Rear3LeftShaftOutput/1(Trq[Nm]___UNIQUE_1)
